simulink library "FSCtrl_cl"  (R2020a)
settings: Solver=VariableStepAuto  StartTime=0.0  StopTime=10.0  RelTol=1e-3
undefined symbols (not defined in the file or in its folder): a, env, FLIGHTCONTROLLER, fltCtrl, initializeBussesFromBlock, pthCtrl1, pthCtrl2, slfCtrl, thr, vhcl, wnch
libraries: simulink x22, angleBtw2Vecs_ul x6, filteredPIDController_ul x5, velocityAngle_ul x4, ctrlAllocMatrix_cl x3, filteredPIDControllerAWGS_ul x3, eulAng2RotMat_ul x3, vrlib x3, alphaBeta_ul x3, gnd2TanRotation_ul x3, pathGeometry_ul x3, filteredPIDControllerAW_ul x2
(part 2 of 3)

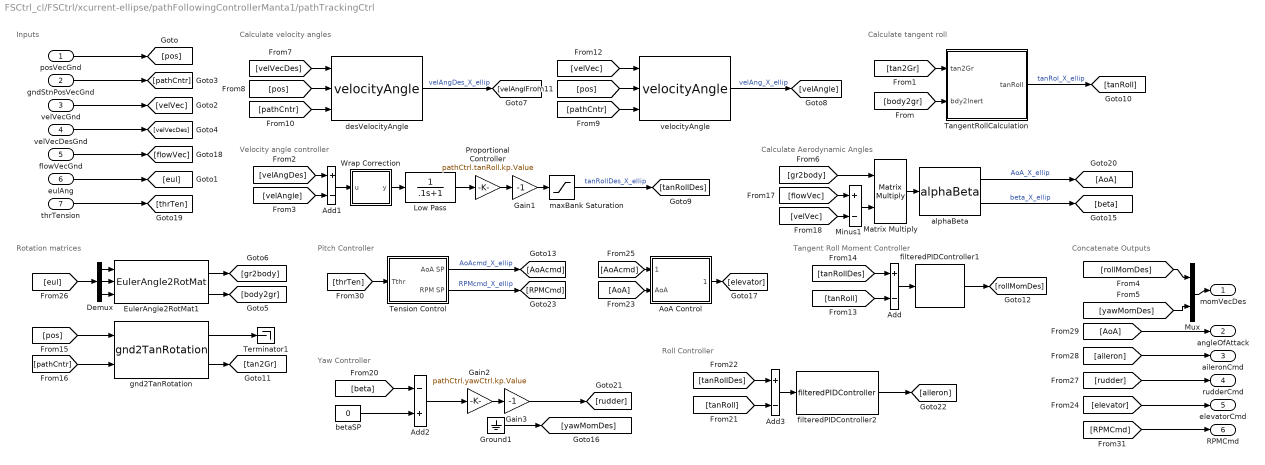
== system FSCtrl_cl/FSCtrl/xcurrent-ellipse/pathFollowingControllerManta1/pathTrackingCtrl ==
  note: Pitch Controller
  note: Calculate Aerodynamic Angles
  note: Yaw Controller
  note: Concatenate Outputs
  note: Tangent Roll Moment Controller
  note: Calculate tangent roll
  note: Calculate velocity angles
  note: Rotation matrices
  note: Inputs
  note: Velocity angle controller
  note: Roll Controller
  posVecGnd : Inport
  gndStnPosVecGnd : Inport  Port=2
  velVecGnd : Inport  Port=3
  velVecDesGnd : Inport  Port=4
  flowVecGnd : Inport  Port=5
  eulAng : Inport  Port=6
  thrTension : Inport  Port=7
  Add : Sum  Inputs=+-
  Add1 : Sum  Inputs=+-
  Add2 : Sum  Inputs=-+
  Add3 : Sum  Inputs=+-
  AoA Control : Subsystem
  Demux : Demux  Outputs=3
  EulerAngle2RotMat1 : eulAng2RotMat_ul/EulerAngle2RotMat  SystemSampleTime=-1  Latency=0  AutoFrameSizeCalculation=off
  Gain1 : Gain  Gain=-1
  Gain2 : Gain  Gain=pathCtrl.yawCtrl.kp.Value
  Gain3 : Gain  Gain=-1
  Ground1 : Ground
  Low Pass : TransferFcn  Denominator=[.1 1]
  Matrix Multiply : Product  Multiplication=Matrix(*)
  Minus1 : Sum  Inputs=+-
  Mux : Mux  Inputs=2
  Proportional Controller : Gain  Gain=pathCtrl.tanRoll.kp.Value
  TangentRollCalculation : Subsystem
  Tension Control : Subsystem
  Terminator1 : Terminator
  Wrap Correction : Subsystem
  alphaBeta : alphaBeta_ul/alphaBeta  SystemSampleTime=-1  Latency=0  AutoFrameSizeCalculation=off
  betaSP : Constant  Value=0
  desVelocityAngle : velocityAngle_ul/velocityAngle  SystemSampleTime=-1  Latency=0  AutoFrameSizeCalculation=off
  filteredPIDController1 : filteredPIDController_ul/filteredPIDController  kp=pathCtrl.rollMoment.kp.Value  ki=0  kd=pathCtrl.rollMoment.kd.Value  Value=pathCtrl.rollMoment.tau.Value  externalReset=none
  filteredPIDController2 : filteredPIDController_ul/filteredPIDController  kp=pathCtrl.rollCtrl.kp.Value  ki=pathCtrl.rollCtrl.ki.Value  kd=pathCtrl.rollCtrl.kd.Value  Value=pathCtrl.rollCtrl.tau.Value  externalReset=none
  gnd2TanRotation : gnd2TanRotation_ul/gnd2TanRotation  SystemSampleTime=-1  Latency=0  AutoFrameSizeCalculation=off
  maxBank Saturation : Saturate  UpperLimit=pathCtrl.maxBank.upperLimit.Value  LowerLimit=pathCtrl.maxBank.lowerLimit.Value
  velocityAngle : velocityAngle_ul/velocityAngle  SystemSampleTime=-1  Latency=0  AutoFrameSizeCalculation=off
  momVecDes : Outport  VectorParamsAs1DForOutWhenUnconnected=off
  angleOfAttack : Outport  Port=2  VectorParamsAs1DForOutWhenUnconnected=off
  aileronCmd : Outport  Port=3  VectorParamsAs1DForOutWhenUnconnected=off
  rudderCmd : Outport  Port=4  VectorParamsAs1DForOutWhenUnconnected=off
  elevatorCmd : Outport  Port=5  VectorParamsAs1DForOutWhenUnconnected=off
  RPMCmd : Outport  Port=6  VectorParamsAs1DForOutWhenUnconnected=off
  wires:
  Ground1/1 -> [yawMomDes]
  Low Pass/1 -> Proportional Controller/1
  Wrap Correction/1(y) -> Low Pass/1
  posVecGnd/1 -> [pos]
  velVecGnd/1 -> [velVec]
  Add/1 -> filteredPIDController1/1
  Proportional Controller/1 -> Gain1/1
  Gain1/1 -> maxBank Saturation/1
  maxBank Saturation/1 -> [tanRollDes]  "tanRollDes_X_ellip"
  Add1/1 -> Wrap Correction/1(u)
  flowVecGnd/1 -> [flowVec]
  [tan2Gr] -> TangentRollCalculation/1(tan2Gr)
  TangentRollCalculation/1(tanRoll) -> [tanRoll]  "tanRol_X_ellip"
  filteredPIDController1/1 -> [rollMomDes]
  Gain2/1 -> Gain3/1
  Minus1/1 -> Matrix Multiply/2
  [velVec] -> Minus1/2
  [flowVec] -> Minus1/1
  Demux/3 -> EulerAngle2RotMat1/3
  Demux/1 -> EulerAngle2RotMat1/1
  Demux/2 -> EulerAngle2RotMat1/2
  EulerAngle2RotMat1/2 -> [body2gr]
  EulerAngle2RotMat1/1 -> [gr2body]
  [body2gr] -> TangentRollCalculation/2(bdy2Inert)
  [gr2body] -> Matrix Multiply/1
  Matrix Multiply/1 -> alphaBeta/1
  alphaBeta/2 -> [beta]  "beta_X_ellip"
  Add2/1 -> Gain2/1
  Mux/1 -> momVecDes/1
  [yawMomDes] -> Mux/2
  gndStnPosVecGnd/1 -> [pathCntr]
  velVecDesGnd/1 -> [velVecDes]
  desVelocityAngle/1 -> [velAngDes]  "velAngDes_X_ellip"
  velocityAngle/1 -> [velAngle]  "velAng_X_ellip"
  [velAngDes] -> Add1/1
  [velAngle] -> Add1/2
  [velVecDes] -> desVelocityAngle/1
  [pos] -> desVelocityAngle/2
  [pathCntr] -> desVelocityAngle/3
  [velVec] -> velocityAngle/1
  [tanRoll] -> Add/2
  [tanRollDes] -> Add/1
  [pos] -> gnd2TanRotation/1
  [pathCntr] -> gnd2TanRotation/2
  gnd2TanRotation/2 -> [tan2Gr]
  gnd2TanRotation/1 -> Terminator1/1
  [rollMomDes] -> Mux/1
  Tension Control/2(RPM SP) -> [RPMCmd]  "RPMcmd_X_ellip"
  AoA Control/1(elvCmd) -> [elevator]
  Tension Control/1(AoA SP) -> [AoAcmd]  "AoAcmd_X_ellip"
  [AoAcmd] -> AoA Control/1(AoA SP)
  [AoA] -> AoA Control/2(AoA)
  eulAng/1 -> [eul]
  thrTension/1 -> [thrTen]
  [eul] -> Demux/1
  [thrTen] -> Tension Control/1(Tthr)
  [pos] -> velocityAngle/2
  [pathCntr] -> velocityAngle/3
  alphaBeta/1 -> [AoA]  "AoA_X_ellip"
  Gain3/1 -> [rudder]
  [beta] -> Add2/1
  betaSP/1 -> Add2/2
  filteredPIDController2/1 -> [aileron]
  [AoA] -> angleOfAttack/1
  [aileron] -> aileronCmd/1
  [rudder] -> rudderCmd/1
  [elevator] -> elevatorCmd/1
  [tanRollDes] -> Add3/1
  [tanRoll] -> Add3/2
  Add3/1 -> filteredPIDController2/1
  [RPMCmd] -> RPMCmd/1

== system FSCtrl_cl/FSCtrl/xcurrent-lemOfBooth/pathFollowingControllerManta/Concatenation ==
  In1 : Inport
  Demux1 : Demux
  Gain : Gain  Gain=pathCtrl.rudderGain.Value
  Mux : Mux
  Out1 : Outport
  wires:
  In1/1 -> Demux1/1
  Mux/1 -> Out1/1
  Demux1/4 -> Gain/1
  Gain/1 -> Mux/4  "rudderCmd"
  Demux1/2 -> Mux/2  "starBrdCmd"
  Demux1/1 -> Mux/1  "portCmd"
  Demux1/3 -> Mux/3  "elevCmd"

== system FSCtrl_cl/FSCtrl/xcurrent-lemOfBooth/pathFollowingControllerManta/Lap Tracking ==
  pathParameter : Inport
  Add2 : Sum
  Compare To Constant1 : simulink/Logic and Bit Operations/Compare To Constant  relop=>=  const=10  OutDataTypeStr=boolean
  Compare To Constant3 : simulink/Logic and Bit Operations/Compare To Constant  relop=<=  const=0.1  OutDataTypeStr=boolean
  Compare To Constant4 : simulink/Logic and Bit Operations/Compare To Constant  relop=>=  const=0.9  OutDataTypeStr=boolean
  Data Type Conversion2 : DataTypeConversion  OutDataTypeStr=double
  Logical Operator1 : Logic  Inputs=4  AllPortsSameDT=off  OutDataTypeStr=boolean
  Memory : Memory  InitialCondition=false
  Memory3 : Memory
  Memory4 : Memory
  Subsystem : Subsystem
  stopwatch : stopwatch_ul/stopwatch  SystemSampleTime=-1  Latency=0  AutoFrameSizeCalculation=off
  lapNum : Outport  VectorParamsAs1DForOutWhenUnconnected=off
  rst : Outport  Port=2  VectorParamsAs1DForOutWhenUnconnected=off
  wires:
  Subsystem/1(realLap) -> Logical Operator1/3  "real"
  Compare To Constant1/1 -> Logical Operator1/4
  Memory/1 -> stopwatch/1, Subsystem/2(rst)
  stopwatch/1 -> Compare To Constant1/1
  pathParameter/1 -> Memory3/1, Compare To Constant3/1, Subsystem/1(S)
  Compare To Constant4/1 -> Logical Operator1/2
  Add2/1 -> Memory4/1, lapNum/1
  Memory4/1 -> Add2/2
  Logical Operator1/1 -> Memory/1, Data Type Conversion2/1, rst/1
  Data Type Conversion2/1 -> Add2/1
  Memory3/1 -> Compare To Constant4/1
  Compare To Constant3/1 -> Logical Operator1/1

== system FSCtrl_cl/FSCtrl/xcurrent-lemOfBooth/pathFollowingControllerManta/Subsystem ==
  posVecGnd : Inport
  Atan1 : Trigonometry  Operator=atan2
  Atan2 : Trigonometry  Operator=atan2
  Gain : Gain  Gain=180/pi
  Gain1 : Gain  Gain=180/pi
  Selector1 : Selector  InputPortWidth=3  IndexOptions=Index vector (dialog)  Indices=1  OutputSizes=1
  Selector2 : Selector  InputPortWidth=3  IndexOptions=Index vector (dialog)  Indices=[1 2]  OutputSizes=1
  Selector3 : Selector  InputPortWidth=3  IndexOptions=Index vector (dialog)  Indices=3  OutputSizes=1
  Selector4 : Selector  InputPortWidth=3  IndexOptions=Index vector (dialog)  Indices=2  OutputSizes=1
  Sqrt1 : Sqrt  SaturateOnIntegerOverflow=on
  Sqrt2 : Sqrt  SaturateOnIntegerOverflow=on
  Square1 : Math  Operator=square  SignedPower=on  SaturateOnIntegerOverflow=on
  Square2 : Math  Operator=square  SignedPower=on  SaturateOnIntegerOverflow=on
  Sum of Elements : Sum  Inputs=+
  Sum of Elements1 : Sum  Inputs=+
  elevationAngle : Outport
  azimuth Angle : Outport  Port=2
  wires:
  Gain1/1 -> azimuth Angle/1
  Selector4/1 -> Atan2/1
  Sqrt2/1 -> Atan2/2
  posVecGnd/1 -> Selector3/1, Selector2/1, Selector4/1, Selector1/1
  Selector1/1 -> Square2/1
  Sum of Elements1/1 -> Sqrt2/1
  Square2/1 -> Sum of Elements1/1
  Atan2/1 -> Gain1/1
  Gain/1 -> elevationAngle/1
  Selector2/1 -> Square1/1
  Atan1/1 -> Gain/1
  Sum of Elements/1 -> Sqrt1/1
  Selector3/1 -> Atan1/1
  Square1/1 -> Sum of Elements/1
  Sqrt1/1 -> Atan1/2

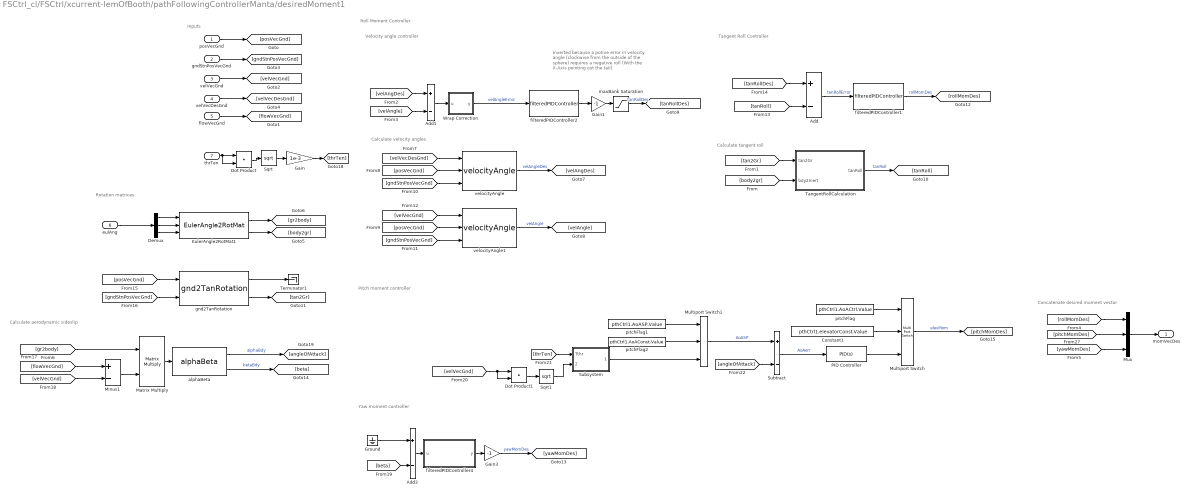
== system FSCtrl_cl/FSCtrl/xcurrent-lemOfBooth/pathFollowingControllerManta/desiredMoment1 ==
  note: Roll Moment Controller
  note: Calculate aerodynamic sideslip
  note: Concatenate desired moment vector
  note: Tangent Roll Controller
  note: Calculate tangent roll
  note: Calculate velocity angles
  note: Rotation matrices
  note: Inputs
  note: Velocity angle controller
  note: Inverted because a potive error
      | in velocity angle (clockwise from the
      | outside of the sphere) requires a negative
      | roll (With the X-Axis pointing out the tail)
  note: Pitch moment controller
  note: Yaw moment controller
  posVecGnd : Inport
  gndStnPosVecGnd : Inport  Port=2
  velVecGnd : Inport  Port=3
  velVecDesGnd : Inport  Port=4
  flowVecGnd : Inport  Port=5
  eulAng : Inport  Port=6
  thrTen : Inport  Port=7
  Add : Sum  Inputs=+-
  Add1 : Sum  Inputs=+-
  Add3 : Sum  Inputs=+-
  Constant1 : Constant  Value=pthCtrl1.elevatorConst.Value
  Demux : Demux  Outputs=3
  Dot Product : DotProduct  InputSameDT=on  OutDataTypeStr=Inherit: Inherit via internal rule
  Dot Product1 : DotProduct  InputSameDT=on  OutDataTypeStr=Inherit: Inherit via internal rule
  EulerAngle2RotMat1 : eulAng2RotMat_ul/EulerAngle2RotMat  SystemSampleTime=-1  Latency=0  AutoFrameSizeCalculation=off
  Gain : Gain  Gain=1e-3
  Gain1 : Gain  Gain=-1
  Gain3 : Gain  Gain=-1
  Ground : Ground
  Matrix Multiply : Product  Multiplication=Matrix(*)
  Minus1 : Sum  Inputs=+-
  Multiport Switch : MultiPortSwitch  DataPortOrder=Specify indices  Inputs=2  DataPortIndices={0,1}
  Multiport Switch1 : MultiPortSwitch  DataPortOrder=Specify indices  Inputs=2  DataPortIndices={0,1}
  Mux : Mux  Inputs=3
  PID Controller : simulink/Continuous/PID Controller  Controller=PID  Form=Parallel  TimeDomain=Continuous-time  UseExternalTs=off  SampleTime=-1  IntegratorMethod=Forward Euler  FilterMethod=Forward Euler  ControllerParametersSource=internal  P=pthCtrl1.pitchMoment.kp.Value  I=pthCtrl1.pitchMoment.ki.Value  D=pthCtrl1.pitchMoment.kd.Value  UseFilter=on  N=pthCtrl1.pitchMoment.tau.Value  TunerSelectOption=Transfer Function Based (PID Tuner App)  InitialConditionSource=internal  InitialConditionForIntegrator=0  InitialConditionForFilter=0  DifferentiatorICPrevScaledInput=0  ExternalReset=none  TrackingMode=off  Kt=1  LimitOutput=off  UpperSaturationLimit=inf  LowerSaturationLimit=-100  LinearizeAsGain=on  AntiWindupMode=clamping  Kb=1  POutMin=[]  POutMax=[]  IOutMin=[]  IOutMax=[]  DOutMin=[]  DOutMax=[]  NOutMin=[]  NOutMax=[]  SumOutMin=[]  SumOutMax=[]  SaturationOutMin=[]  SaturationOutMax=[]  PParamMin=[]  PParamMax=[]  IParamMin=[]  IParamMax=[]  DParamMin=[]  DParamMax=[]  NParamMin=[]  NParamMax=[]  KbParamMin=[]  KbParamMax=[]  KtParamMin=[]  KtParamMax=[]  KbOutMin=[]  KbOutMax=[]  KtOutMin=[]  KtOutMax=[]  IntegratorOutMin=[]  IntegratorOutMax=[]  FilterOutMin=[]  FilterOutMax=[]  SumI1OutMin=[]  SumI1OutMax=[]  SumI2OutMin=[]  SumI2OutMax=[]  SumI3OutMin=[]  SumI3OutMax=[]  SumI4OutMin=[]  SumI4OutMax=[]  SumDOutMin=[]  SumDOutMax=[]  DifferentiatorOutMin=[]  DifferentiatorOutMax=[]  FilterDiffOutCoefMin=[]  FilterDiffOutCoefMax=[]  ReciprocalOutMin=[]  ReciprocalOutMax=[]  SumDenOutMin=[]  SumDenOutMax=[]  SumNumOutMin=[]  SumNumOutMax=[]  DivideOutMin=[]  DivideOutMax=[]  UdiffTsProdOutMin=[]  UdiffTsProdOutMax=[]  NTsProdOutMin=[]  NTsProdOutMax=[]  UintegralTsProdOutMin=[]  UintegralTsProdOutMax=[]  UngainTsProdOutMin=[]  UngainTsProdOutMax=[]  IntegratorContinuousStateAttributes=''  IntegratorStateMustResolveToSignalObject=off  IntegratorRTWStateStorageClass=Auto  FilterContinuousStateAttributes=''  FilterStateMustResolveToSignalObject=off  FilterRTWStateStorageClass=Auto  ParallelPVariant=InternalParameters  IdealPVariant=Disabled  IVariant=InternalParameters  DVariant=InternalParameters  IntegratorVariant=Continuous  SatVariant=Disabled  AWVariant=Passthrough  PCopyVariant=Disabled  TRVariant=Disabled  FdbkBlocksVariant=Forward  IdealPFdbkVariant=Disabled  SatFdbkVariant=Disabled  DerivativeFilterVariant=ContFilter  NVariant=InternalParameters  NCopyVariant=Disabled  FilterICVariant=InternalICsFilter  IntegratorICVariant=InternalICs  ExternalResetVariant=Disabled  TRSumVariant=Passthrough  SumFdbkVariant=Disabled  SumVariant=Sum_PID  TsampFilterVariant=InternalTs  TsampNgainVariant=Passthrough  TsampIntegralVariant=Passthrough
  Sqrt : Sqrt  SaturateOnIntegerOverflow=on
  Sqrt1 : Sqrt  SaturateOnIntegerOverflow=on
  Subsystem : Subsystem
  Subtract : Sum  Inputs=+-
  TangentRollCalculation : Subsystem
  Terminator1 : Terminator
  Wrap Correction : Subsystem
  alphaBeta : alphaBeta_ul/alphaBeta  SystemSampleTime=-1  Latency=0  AutoFrameSizeCalculation=off
  filteredPIDController1 : filteredPIDController_ul/filteredPIDController  kp=pathCtrl.rollMoment.kp.Value  ki=0  kd=pathCtrl.rollMoment.kd.Value  Value=pathCtrl.rollMoment.tau.Value  externalReset=none
  filteredPIDController2 : filteredPIDController_ul/filteredPIDController  kp=pathCtrl.tanRoll.kp.Value  ki=pathCtrl.tanRoll.ki.Value  kd=pathCtrl.tanRoll.kd.Value  Value=pathCtrl.tanRoll.tau.Value  externalReset=none
  filteredPIDController4 : Subsystem  mask{kp=pthCtrl1.yawMoment.kp.Value, ki=0, kd=pathCtrl.yawMoment.kd.Value, Value=pathCtrl.yawMoment.tau.Value, externalReset=none}
      mask prompts: kp "Proportional Gain, kp"; ki "Integral Gain, ki"; kd "Derivative Gain, kd"; Value "Time Constant, s"; externalReset "External reset:"
      mask init:
      | initfcn
      mask TypeOptions kp: kp/Gain
      mask TypeOptions ki: ki/Gain
      mask TypeOptions kd: kd/Gain
      mask TypeOptions Value: tau/Value
      mask TypeOptions externalReset: none | rising | falling | either | level | level hold
  gnd2TanRotation : gnd2TanRotation_ul/gnd2TanRotation  SystemSampleTime=-1  Latency=0  AutoFrameSizeCalculation=off
  maxBank Saturation : Saturate  UpperLimit=pathCtrl.maxBank.upperLimit.Value  LowerLimit=pathCtrl.maxBank.lowerLimit.Value
  pitchFlag : Constant  Value=pthCtrl1.AoACtrl.Value
  pitchFlag1 : Constant  Value=pthCtrl1.AoASP.Value
  pitchFlag2 : Constant  Value=pthCtrl1.AoAConst.Value
  velocityAngle : velocityAngle_ul/velocityAngle  SystemSampleTime=-1  Latency=0  AutoFrameSizeCalculation=off
  velocityAngle1 : velocityAngle_ul/velocityAngle  SystemSampleTime=-1  Latency=0  AutoFrameSizeCalculation=off
  momVecDes : Outport  VectorParamsAs1DForOutWhenUnconnected=off
  wires:
  filteredPIDController1/1 -> [rollMomDes]  "rollMomDes"
  [rollMomDes] -> Mux/1
  Wrap Correction/1(y) -> filteredPIDController2/1  "velAngleError"
  posVecGnd/1 -> [posVecGnd]
  velVecGnd/1 -> [velVecGnd]
  Add/1 -> filteredPIDController1/1  "tanRollError"
  Gain1/1 -> maxBank Saturation/1
  maxBank Saturation/1 -> [tanRollDes]  "tanRollDes"
  Add1/1 -> Wrap Correction/1(u)
  flowVecGnd/1 -> [flowVecGnd]
  [tan2Gr] -> TangentRollCalculation/1(tan2Gr)
  TangentRollCalculation/1(tanRoll) -> [tanRoll]  "tanRoll"
  Minus1/1 -> Matrix Multiply/2
  [velVecGnd] -> Minus1/2
  [flowVecGnd] -> Minus1/1
  eulAng/1 -> Demux/1
  Demux/2 -> EulerAngle2RotMat1/2
  EulerAngle2RotMat1/2 -> [body2gr]
  EulerAngle2RotMat1/1 -> [gr2body]
  [body2gr] -> TangentRollCalculation/2(bdy2Inert)
  [gr2body] -> Matrix Multiply/1
  Matrix Multiply/1 -> alphaBeta/1
  alphaBeta/2 -> [beta]  "betaBdy"
  alphaBeta/1 -> [angleOfAttack]  "alphaBdy"
  gndStnPosVecGnd/1 -> [gndStnPosVecGnd]
  velVecDesGnd/1 -> [velVecDesGnd]
  velocityAngle/1 -> [velAngDes]  "velAngleDes"
  velocityAngle1/1 -> [velAngle]  "velAngle"
  [velAngDes] -> Add1/1
  [velAngle] -> Add1/2
  [velVecDesGnd] -> velocityAngle/1
  [posVecGnd] -> velocityAngle/2
  [posVecGnd] -> velocityAngle1/2
  [gndStnPosVecGnd] -> velocityAngle/3
  [gndStnPosVecGnd] -> velocityAngle1/3
  [velVecGnd] -> velocityAngle1/1
  [tanRoll] -> Add/2
  [tanRollDes] -> Add/1
  [posVecGnd] -> gnd2TanRotation/1
  [gndStnPosVecGnd] -> gnd2TanRotation/2
  gnd2TanRotation/2 -> [tan2Gr]
  gnd2TanRotation/1 -> Terminator1/1
  [yawMomDes] -> Mux/3
  filteredPIDController2/1 -> Gain1/1
  [beta] -> Add3/2
  Ground/1 -> Add3/1
  Add3/1 -> filteredPIDController4/1(u)
  filteredPIDController4/1(y) -> Gain3/1
  Subsystem/1(AoA SP) -> Multiport Switch1/3
  [thrTen] -> Subsystem/1(Tthr)
  pitchFlag1/1 -> Multiport Switch1/1
  pitchFlag2/1 -> Multiport Switch1/2
  [pitchMomDes] -> Mux/2
  Gain3/1 -> [yawMomDes]  "yawMomDes"
  Multiport Switch/1 -> [pitchMomDes]  "elevMom"
  pitchFlag/1 -> Multiport Switch/1
  [angleOfAttack] -> Subtract/2
  Constant1/1 -> Multiport Switch/2
  PID Controller/1 -> Multiport Switch/3
  Subtract/1 -> PID Controller/1  "AoAerr"
  thrTen/1 -> Dot Product/2, Dot Product/1
  Sqrt/1 -> Gain/1
  Dot Product/1 -> Sqrt/1
  Gain/1 -> [thrTen]
  [velVecGnd] -> Dot Product1/2, Dot Product1/1
  Sqrt1/1 -> Subsystem/2(vAppSqr)
  Dot Product1/1 -> Sqrt1/1
  Demux/1 -> EulerAngle2RotMat1/1
  Demux/3 -> EulerAngle2RotMat1/3
  Mux/1 -> momVecDes/1
  Multiport Switch1/1 -> Subtract/1  "AoASP"

== system FSCtrl_cl/FSCtrl/non-xcurrent/LaRController/desiredMoment/TangentRollCalculation ==
  note: Angle between body X and tangent Z
  note: Inverted because the right wing
      | being <90deg from Local down
      | is a negative roll about the +X axis
  note: Angle between body Y and tangent Z
  note: Measuring tangent roll as the opposite
      | of the angle between the Body Y axis
      | and the tangent plane
  tan2Gr : Inport
  bdy2Inert : Inport  Port=2
  Constant1 : Constant  Value=pi/2
  Constant2 : Constant  Value=pi/2
  Constant3 : Constant  Value=[0 1 0]'
  Constant4 : Constant  Value=[0 0 1]'
  Constant5 : Constant  Value=[1 0 0]'
  Constant6 : Constant  Value=[0 0 1]'
  Gain : Gain  Gain=-1
  Matrix Multiply{,1..3} (4 alike) : Product  Multiplication=Matrix(*)
  Subtract : Sum  Inputs=+-
  Subtract1 : Sum  Inputs=+-
  Terminator : Terminator
  angleBtw2DVecs : angleBtw2Vecs_ul/angleBtw2DVecs  SystemSampleTime=-1  Latency=0  AutoFrameSizeCalculation=off
  angleBtw2DVecs1 : Subsystem
  tanRoll : Outport  VectorParamsAs1DForOutWhenUnconnected=off
  wires:
  Constant5/1 -> Matrix Multiply2/2
  angleBtw2DVecs1/1(angle) -> Subtract1/2
  Constant1/1 -> Subtract1/1
  Matrix Multiply3/1 -> angleBtw2DVecs1/1(vec1)
  Constant6/1 -> Matrix Multiply3/2
  Matrix Multiply2/1 -> angleBtw2DVecs1/2(vec2)
  tan2Gr/1 -> Matrix Multiply1/1, Matrix Multiply3/1
  Subtract1/1 -> Terminator/1  "tanPitch"
  bdy2Inert/1 -> Matrix Multiply/1, Matrix Multiply2/1
  Gain/1 -> tanRoll/1  "tanRoll"
  Subtract/1 -> Gain/1
  Matrix Multiply/1 -> angleBtw2DVecs/2
  Constant4/1 -> Matrix Multiply1/2
  Matrix Multiply1/1 -> angleBtw2DVecs/1
  Constant2/1 -> Subtract/1
  angleBtw2DVecs/1 -> Subtract/2
  Constant3/1 -> Matrix Multiply/2

== system FSCtrl_cl/FSCtrl/non-xcurrent/LaRController/winchController/vectorMagnitude ==
  Vec : Inport
  Reshape4 : Reshape
  Sqrt : Sqrt  SaturateOnIntegerOverflow=on
  Square : Math  Operator=square  SaturateOnIntegerOverflow=on
  Sum of Elements : Sum  Inputs=+
  Mag : Outport
  wires:
  Reshape4/1 -> Mag/1
  Vec/1 -> Square/1
  Sum of Elements/1 -> Sqrt/1
  Square/1 -> Sum of Elements/1
  Sqrt/1 -> Reshape4/1

== system FSCtrl_cl/FSCtrl/xcurrent-ellipse/pathFollowingControllerManta1/Lap Tracking/Subsystem ==
  note: this may have issues when it starts up after a hiatus for a multicycle spool in
      | Hopefully, it will work because the reasonable spooling ranges are already set
  S : Inport
  rst : Inport  Port=2
  AND : Logic  AllPortsSameDT=off  OutDataTypeStr=boolean
  Add : Sum
  Cast To Double : DataTypeConversion  OutDataTypeStr=double
  Compare To Constant : simulink/Logic and Bit Operations/Compare To Constant  relop=>=  const=.99  OutDataTypeStr=boolean
  Compare To Constant1 : simulink/Logic and Bit Operations/Compare To Constant  relop=<=  const=.01  OutDataTypeStr=boolean
  Divide : Product  Inputs=**
  Divide1 : Product  Inputs=**
  Gain : Gain  Gain=-1
  Max : MinMax  Function=max  Inputs=2
  Max1 : MinMax  Inputs=2
  One : Constant  OutDataTypeStr=Inherit: Inherit via back propagation
  Power : Math  Operator=pow  SaturateOnIntegerOverflow=on
  Power1 : Math  Operator=pow  SaturateOnIntegerOverflow=on
  memoryIC1 : Memory  InitialCondition=1
  memoryIC=0 : Memory
  memoryIC=1 : Memory  InitialCondition=1
  realLap : Outport
  wires:
  memoryIC1/1 -> Power/1
  memoryIC=1/1 -> Power1/1
  [zeroIfReset] -> Power1/2
  memoryIC=0/1 -> Divide1/1
  Divide1/1 -> Max/2
  [zeroIfReset] -> Divide1/2
  [zeroIfReset] -> Power/2
  [zeroIfReset] -> Divide/2
  AND/1 -> realLap/1
  Compare To Constant1/1 -> AND/2
  Compare To Constant/1 -> AND/1
  Cast To Double/1 -> Gain/1
  Power1/1 -> Max1/2
  Power/1 -> Max1/1
  Max/1 -> Compare To Constant/1, memoryIC=0/1
  Divide/1 -> Max/1
  One/1 -> Add/2
  Add/1 -> [zeroIfReset]
  Gain/1 -> Add/1
  S/1 -> memoryIC1/1, Divide/1
  rst/1 -> Cast To Double/1
  Max1/1 -> memoryIC=1/1, Compare To Constant1/1

== system FSCtrl_cl/FSCtrl/xcurrent-ellipse/pathFollowingControllerManta1/courseFollowManta/GoldenSectionPathSearch ==
  lastKnownS : Inport
  pathParams : Inport  Port=2
  currentPos : Inport  Port=3
  pathCntr : Inport  Port=4
  From11 : From  Commented=on  GotoTag=geomParams
  From27 : From  Commented=on  GotoTag=pathCntr
  From28 : From  Commented=on  GotoTag=pos
  From30 : From  Commented=on  GotoTag=sPrev
  GoldenSectionMATLAB : MATLAB Function  Commented=on  TreatAsAtomicUnit=on  mask{geomFunc=pathCtrl, searchWidth=0.1, pathVarTol=1e-5}
  GoldenSectionSimulink : Subsystem
  Goto1 : Goto  Commented=on  GotoTag=sStar
  sStar : Outport  InitialOutput=pathCtrl.initPathVar.Value  VectorParamsAs1DForOutWhenUnconnected=off
  wires:
  GoldenSectionSimulink/1(Out1) -> [sStar]
  [sPrev] -> GoldenSectionSimulink/4(sPrev)
  [pathCntr] -> GoldenSectionSimulink/3(cntrPtPosVec)
  [geomParams] -> GoldenSectionSimulink/2(geomParams)
  [pos] -> GoldenSectionSimulink/1(posVecGnd)
  [sStar] -> sStar/1
  lastKnownS/1 -> [sPrev]
  From27/1 -> GoldenSectionMATLAB/3(pathCntrPosVecGnd)
  From30/1 -> GoldenSectionMATLAB/2(sPrev)
  From28/1 -> GoldenSectionMATLAB/1(posVec)
  From11/1 -> GoldenSectionMATLAB/4(geomParams)
  GoldenSectionMATLAB/1(sNext) -> Goto1/1
  pathCntr/1 -> [pathCntr]
  pathParams/1 -> [geomParams]
  currentPos/1 -> [pos]

== system FSCtrl_cl/FSCtrl/xcurrent-ellipse/pathFollowingControllerManta1/courseFollowManta/Overwrite Radius ==
  note: subsystem overwrites the 5th basis parameter with the current radius
      | so that the downstream blocks calculate the path geomatry at the current radius.
  pathParamsIn : Inport
  positionVec : Inport  Port=2
  gndStnPos : Inport  Port=3
  Add : Sum  Inputs=+-
  Assignment : Assignment  NumberOfDimensions=2  DiagnosticForDimensions=Warning  IndexOptions=Index vector (dialog),Assign all  Indices=5,5  OutputSizes=1,1
  Dot Product : DotProduct  InputSameDT=on  OutDataTypeStr=Inherit: Inherit via internal rule
  Sqrt : Sqrt  SaturateOnIntegerOverflow=on
  pathParamsOut : Outport  VectorParamsAs1DForOutWhenUnconnected=off
  wires:
  gndStnPos/1 -> Add/2
  positionVec/1 -> Add/1
  pathParamsIn/1 -> Assignment/1
  Sqrt/1 -> Assignment/2
  Assignment/1 -> pathParamsOut/1
  Dot Product/1 -> Sqrt/1
  Add/1 -> Dot Product/1, Dot Product/2

== system FSCtrl_cl/FSCtrl/xcurrent-ellipse/pathFollowingControllerManta1/courseFollowManta/saturatedWeightedAverage ==
  note: 0 if error=0
      | 1 if error>=upper_lim
  note: from mask
  note: errorVar must be positive
  "errorVar " : Inport
  tangVector : Inport  Port=2
  "perpVector " : Inport  Port=3
  Add : Sum  Commented=on  Inputs=+-
  Add1 : Sum  Commented=on
  Add2 : Sum  Inputs=+-
  Add3 : Sum
  Constant : Constant  Value=error_upper_lim
  Constant1 : Constant  Commented=on  Value=a
  Constant2 : Constant  Commented=on
  Constant4 : Constant
  Divide : Product  Inputs=*/
  Exp : Math  Commented=on  SignedPower=on  SaturateOnIntegerOverflow=on
  From : From  Commented=on  GotoTag=errorVar
  From1 : From  Commented=on  GotoTag=perpVec
  From2 : From  Commented=on  GotoTag=tangVec
  Gain : Gain  Commented=on  Gain=-1
  Multiply : Product  Commented=on
  Multiply1 : Product  Commented=on
  Multiply2 : Product  Commented=on
  Multiply3 : Product
  Multiply5 : Product
  Saturation : Saturate  UpperLimit=1  LowerLimit=0
  "velVectorDes " : Outport  VectorParamsAs1DForOutWhenUnconnected=off
  wires:
  tangVector/1 -> [tangVector]
  Constant1/1 -> Gain/1
  Gain/1 -> Multiply1/1
  Multiply1/1 -> Exp/1
  Exp/1 -> Multiply/1, Add/2  "e^(-a*errorVar) 0 if error=inf 1 if error=0"
  Constant2/1 -> Add/1
  Add/1 -> Multiply2/1  "1-e^(-a*errorVar) 0 if error=0 1 if error=inf"
  "errorVar "/1 -> [errorVar]
  "perpVector "/1 -> [perpVector]
  From/1 -> Multiply1/2
  Multiply2/1 -> Add1/1
  Multiply/1 -> Add1/2
  From1/1 -> Multiply2/2
  From2/1 -> Multiply/2
  Constant4/1 -> Add2/1
  Saturation/1 -> Multiply3/1, Add2/2
  Add3/1 -> "velVectorDes "/1
  Multiply3/1 -> Add3/2
  Multiply5/1 -> Add3/1
  Add2/1 -> Multiply5/1  "0 if error>=upper_lim 1 if error=inf"
  [errorVar] -> Divide/1
  Constant/1 -> Divide/2
  Divide/1 -> Saturation/1
  [tangVector] -> Multiply5/2
  [perpVector] -> Multiply3/2

== system FSCtrl_cl/FSCtrl/xcurrent-ellipse/pathFollowingControllerManta1/pathTrackingCtrl/AoA Control ==
  AoA SP : Inport
  AoA : Inport  Port=2
  Constant1 : Constant  Value=pathCtrl.elevatorConst.Value
  Constant3 : Constant  Value=pathCtrl.elevCtrl.kp.Value
  Constant4 : Constant  Value=pathCtrl.elevCtrl.ki.Value
  Constant5 : Constant  Value=pathCtrl.elevCtrl.kd.Value
  Constant6 : Constant  Value=pathCtrl.elevCtrl.tau.Value
  Multiport Switch : MultiPortSwitch  DataPortOrder=Specify indices  Inputs=2  DataPortIndices={0,1}
  Mux : Mux
  Saturation : Saturate  UpperLimit=pathCtrl.elevCtrlMax.upperLimit.Value  LowerLimit=pathCtrl.elevCtrlMax.lowerLimit.Value
  Subtract : Sum  Inputs=-+
  filteredPIDControllerAWGS : filteredPIDControllerAWGS_ul/filteredPIDControllerAWGS  cmax=pathCtrl.elevCtrlMax.upperLimit.Value  cmin=pathCtrl.elevCtrlMax.lowerLimit.Value
  pitchFlag : Constant  Value=pathCtrl.AoACtrl.Value
  elvCmd : Outport
  wires:
  Constant6/1 -> Mux/4
  Constant5/1 -> Mux/3
  Constant4/1 -> Mux/2
  Constant3/1 -> Mux/1
  Mux/1 -> [gains]
  [gains] -> filteredPIDControllerAWGS/2
  filteredPIDControllerAWGS/1 -> Multiport Switch/3
  Subtract/1 -> filteredPIDControllerAWGS/1
  Saturation/1 -> elvCmd/1
  Multiport Switch/1 -> Saturation/1
  AoA SP/1 -> Subtract/1
  pitchFlag/1 -> Multiport Switch/1
  Constant1/1 -> Multiport Switch/2
  AoA/1 -> Subtract/2

== system FSCtrl_cl/FSCtrl/xcurrent-ellipse/pathFollowingControllerManta1/pathTrackingCtrl/TangentRollCalculation ==
  note: Measuring tangent roll as the opposite
      | of the angle between the Body Y axis
      | and the tangent plane
  note: Angle between body Y and tangent Z
  note: Inverted because the right wing
      | being <90deg from Local down
      | is a negative roll about the +X axis
  note: Angle between body X and tangent Z
  tan2Gr : Inport
  bdy2Inert : Inport  Port=2
  Constant1 : Constant  Value=pi/2
  Constant2 : Constant  Value=pi/2
  Constant3 : Constant  Value=[0 1 0]'
  Constant4 : Constant  Value=[0 0 1]'
  Constant5 : Constant  Value=[1 0 0]'
  Constant6 : Constant  Value=[0 0 1]'
  Gain : Gain  Gain=-1
  Matrix Multiply{,1..3} (4 alike) : Product  Multiplication=Matrix(*)
  Subtract : Sum  Inputs=+-
  Subtract1 : Sum  Inputs=+-
  Terminator : Terminator
  angleBtw2DVecs : angleBtw2Vecs_ul/angleBtw2DVecs  SystemSampleTime=-1  Latency=0  AutoFrameSizeCalculation=off
  angleBtw2DVecs1 : Subsystem
  tanRoll : Outport  VectorParamsAs1DForOutWhenUnconnected=off
  wires:
  Subtract/1 -> Gain/1
  Constant3/1 -> Matrix Multiply/2
  angleBtw2DVecs/1 -> Subtract/2
  Constant2/1 -> Subtract/1
  Matrix Multiply1/1 -> angleBtw2DVecs/1
  Constant4/1 -> Matrix Multiply1/2
  Matrix Multiply/1 -> angleBtw2DVecs/2
  Gain/1 -> tanRoll/1  "tanRoll"
  bdy2Inert/1 -> Matrix Multiply2/1, Matrix Multiply/1
  Subtract1/1 -> Terminator/1  "tanPitch"
  tan2Gr/1 -> Matrix Multiply3/1, Matrix Multiply1/1
  Matrix Multiply2/1 -> angleBtw2DVecs1/2(vec2)
  Constant6/1 -> Matrix Multiply3/2
  Matrix Multiply3/1 -> angleBtw2DVecs1/1(vec1)
  Constant1/1 -> Subtract1/1
  angleBtw2DVecs1/1(angle) -> Subtract1/2
  Constant5/1 -> Matrix Multiply2/2

== system FSCtrl_cl/FSCtrl/xcurrent-ellipse/pathFollowingControllerManta1/pathTrackingCtrl/Tension Control ==
  Tthr : Inport
  Compare To Constant : simulink/Logic and Bit Operations/Compare To Constant  relop===  const=1  OutDataTypeStr=boolean
  Constant : Constant  Value=pathCtrl.TmaxCtrl.Value
  Multiport Switch2 : MultiPortSwitch  DataPortOrder=Specify indices  Inputs=2  DataPortIndices={0,1}
  pitchFlag1 : Constant  Value=pathCtrl.AoASP.Value
  pitchFlag2 : Constant  Value=pathCtrl.AoAConst.Value
  tensionLimitAoA : tensionLimitAoA_cl/tensionLimitAoA  SystemSampleTime=-1  VariantControl=pathCtrl.TmaxCtrl.Value == 1  Latency=0  AutoFrameSizeCalculation=off
  AoA SP : Outport
  RPM SP : Outport  Port=2
  wires:
  [RPM1] -> RPM SP/1
  Compare To Constant/1 -> tensionLimitAoA/Enable
  Constant/1 -> Compare To Constant/1
  Tthr/1 -> tensionLimitAoA/1
  tensionLimitAoA/1 -> [AoA1]
  tensionLimitAoA/2 -> [RPM1]
  pitchFlag1/1 -> Multiport Switch2/1
  pitchFlag2/1 -> Multiport Switch2/2
  [AoA1] -> Multiport Switch2/3
  Multiport Switch2/1 -> AoA SP/1

== system FSCtrl_cl/FSCtrl/xcurrent-ellipse/pathFollowingControllerManta1/pathTrackingCtrl/Wrap Correction ==
  note: output = mod(input-pi,2*pi)-pi
      | wraps output to -pi to pi
      |
      | ex) 1.5*pi will become -.5pi
      | 	and -1.5pi will become .5pi
      |
      | to visualize, plot the fuction above
  u : Inport
  Add1 : Sum  Inputs=+-
  Add2 : Sum  Inputs=+-
  Constant1 : Constant  Value=pi
  Constant2 : Constant  Value=2*pi
  Constant3 : Constant  Value=pi
  Mod : Math  Operator=mod  SignedPower=on  SaturateOnIntegerOverflow=on
  y : Outport  VectorParamsAs1DForOutWhenUnconnected=off
  wires:
  u/1 -> Add1/1
  Constant1/1 -> Add1/2
  Add1/1 -> Mod/1
  Constant2/1 -> Mod/2
  Mod/1 -> Add2/1  "always_pos"
  Constant3/1 -> Add2/2
  Add2/1 -> y/1

== system FSCtrl_cl/FSCtrl/xcurrent-lemOfBooth/pathFollowingControllerManta/Lap Tracking/Subsystem ==
  note: this may have issues when it starts up after a hiatus for a multicycle spool in
      | Hopefully, it will work because the reasonable spooling ranges are already set
  S : Inport
  rst : Inport  Port=2
  AND : Logic  AllPortsSameDT=off  OutDataTypeStr=boolean
  Add : Sum
  Cast To Double : DataTypeConversion  OutDataTypeStr=double
  Compare To Constant : simulink/Logic and Bit Operations/Compare To Constant  relop=>=  const=.99  OutDataTypeStr=boolean
  Compare To Constant1 : simulink/Logic and Bit Operations/Compare To Constant  relop=<=  const=.01  OutDataTypeStr=boolean
  Divide : Product  Inputs=**
  Divide1 : Product  Inputs=**
  Gain : Gain  Gain=-1
  Max : MinMax  Function=max  Inputs=2
  Max1 : MinMax  Inputs=2
  One : Constant  OutDataTypeStr=Inherit: Inherit via back propagation
  Power : Math  Operator=pow  SaturateOnIntegerOverflow=on
  Power1 : Math  Operator=pow  SaturateOnIntegerOverflow=on
  memoryIC1 : Memory  InitialCondition=1
  memoryIC=0 : Memory
  memoryIC=1 : Memory  InitialCondition=1
  realLap : Outport
  wires:
  memoryIC1/1 -> Power/1
  memoryIC=1/1 -> Power1/1
  [zeroIfReset] -> Power1/2
  memoryIC=0/1 -> Divide1/1
  Divide1/1 -> Max/2
  [zeroIfReset] -> Divide1/2
  [zeroIfReset] -> Power/2
  [zeroIfReset] -> Divide/2
  AND/1 -> realLap/1
  Compare To Constant1/1 -> AND/2
  Compare To Constant/1 -> AND/1
  Cast To Double/1 -> Gain/1
  Power1/1 -> Max1/2
  Power/1 -> Max1/1
  Max/1 -> Compare To Constant/1, memoryIC=0/1
  Divide/1 -> Max/1
  One/1 -> Add/2
  Add/1 -> [zeroIfReset]
  Gain/1 -> Add/1
  S/1 -> memoryIC1/1, Divide/1
  rst/1 -> Cast To Double/1
  Max1/1 -> memoryIC=1/1, Compare To Constant1/1

== system FSCtrl_cl/FSCtrl/xcurrent-lemOfBooth/pathFollowingControllerManta/desiredMoment1/Subsystem ==
  Tthr : Inport
  vAppSqr : Inport  Port=2
  Add : Sum  Inputs=+-
  Constant : Constant  Value=pthCtrl1.Tmax.Value
  Divide : Product  Inputs=*/
  PID Controller : simulink/Continuous/PID Controller  Controller=PID  Form=Parallel  TimeDomain=Continuous-time  UseExternalTs=off  SampleTime=-1  IntegratorMethod=Forward Euler  FilterMethod=Forward Euler  ControllerParametersSource=internal  P=pthCtrl1.alphaCtrl.kp.Value  I=pthCtrl1.alphaCtrl.ki.Value  D=pthCtrl1.alphaCtrl.kd.Value  UseFilter=on  N=pthCtrl1.alphaCtrl.tau.Value  TunerSelectOption=Transfer Function Based (PID Tuner App)  InitialConditionSource=internal  InitialConditionForIntegrator=0  InitialConditionForFilter=0  DifferentiatorICPrevScaledInput=0  ExternalReset=none  TrackingMode=off  Kt=1  LimitOutput=on  UpperSaturationLimit=pthCtrl1.AoAConst.Value  LowerSaturationLimit=pthCtrl1.AoAmin.Value  LinearizeAsGain=on  AntiWindupMode=clamping  Kb=1  POutMin=[]  POutMax=[]  IOutMin=[]  IOutMax=[]  DOutMin=[]  DOutMax=[]  NOutMin=[]  NOutMax=[]  SumOutMin=[]  SumOutMax=[]  SaturationOutMin=[]  SaturationOutMax=[]  PParamMin=[]  PParamMax=[]  IParamMin=[]  IParamMax=[]  DParamMin=[]  DParamMax=[]  NParamMin=[]  NParamMax=[]  KbParamMin=[]  KbParamMax=[]  KtParamMin=[]  KtParamMax=[]  KbOutMin=[]  KbOutMax=[]  KtOutMin=[]  KtOutMax=[]  IntegratorOutMin=[]  IntegratorOutMax=[]  FilterOutMin=[]  FilterOutMax=[]  SumI1OutMin=[]  SumI1OutMax=[]  SumI2OutMin=[]  SumI2OutMax=[]  SumI3OutMin=[]  SumI3OutMax=[]  SumI4OutMin=[]  SumI4OutMax=[]  SumDOutMin=[]  SumDOutMax=[]  DifferentiatorOutMin=[]  DifferentiatorOutMax=[]  FilterDiffOutCoefMin=[]  FilterDiffOutCoefMax=[]  ReciprocalOutMin=[]  ReciprocalOutMax=[]  SumDenOutMin=[]  SumDenOutMax=[]  SumNumOutMin=[]  SumNumOutMax=[]  DivideOutMin=[]  DivideOutMax=[]  UdiffTsProdOutMin=[]  UdiffTsProdOutMax=[]  NTsProdOutMin=[]  NTsProdOutMax=[]  UintegralTsProdOutMin=[]  UintegralTsProdOutMax=[]  UngainTsProdOutMin=[]  UngainTsProdOutMax=[]  IntegratorContinuousStateAttributes=''  IntegratorStateMustResolveToSignalObject=off  IntegratorRTWStateStorageClass=Auto  FilterContinuousStateAttributes=''  FilterStateMustResolveToSignalObject=off  FilterRTWStateStorageClass=Auto  ParallelPVariant=InternalParameters  IdealPVariant=Disabled  IVariant=InternalParameters  DVariant=InternalParameters  IntegratorVariant=Continuous  SatVariant=Enabled  AWVariant=ContClampingParallel  PCopyVariant=Disabled  TRVariant=Disabled  FdbkBlocksVariant=Forward  IdealPFdbkVariant=Disabled  SatFdbkVariant=Disabled  DerivativeFilterVariant=ContFilter  NVariant=InternalParameters  NCopyVariant=Disabled  FilterICVariant=InternalICsFilter  IntegratorICVariant=InternalICs  ExternalResetVariant=Disabled  TRSumVariant=Passthrough  SumFdbkVariant=Disabled  SumVariant=Sum_PID  TsampFilterVariant=InternalTs  TsampNgainVariant=Passthrough  TsampIntegralVariant=Passthrough
  AoA SP : Outport
  wires:
  Divide/1 -> PID Controller/1  "TenErrNorm"
  Constant/1 -> Add/1  "maxTension"
  PID Controller/1 -> AoA SP/1
  Add/1 -> Divide/1  "TenErr"
  vAppSqr/1 -> Divide/2
  Tthr/1 -> Add/2  "thrTen"

== system FSCtrl_cl/FSCtrl/xcurrent-lemOfBooth/pathFollowingControllerManta/desiredMoment1/TangentRollCalculation ==
  note: Measuring tangent roll as the opposite
      | of the angle between the Body Y axis
      | and the tangent plane
  note: Angle between body Y and tangent Z
  note: Inverted because the right wing
      | being <90deg from Local down
      | is a negative roll about the +X axis
  note: Angle between body X and tangent Z
  tan2Gr : Inport
  bdy2Inert : Inport  Port=2
  Constant1 : Constant  Value=pi/2
  Constant2 : Constant  Value=pi/2
  Constant3 : Constant  Value=[0 1 0]'
  Constant4 : Constant  Value=[0 0 1]'
  Constant5 : Constant  Value=[1 0 0]'
  Constant6 : Constant  Value=[0 0 1]'
  Gain : Gain  Gain=-1
  Matrix Multiply{,1..3} (4 alike) : Product  Multiplication=Matrix(*)
  Subtract : Sum  Inputs=+-
  Subtract1 : Sum  Inputs=+-
  Terminator : Terminator
  angleBtw2DVecs : angleBtw2Vecs_ul/angleBtw2DVecs  SystemSampleTime=-1  Latency=0  AutoFrameSizeCalculation=off
  angleBtw2DVecs1 : Subsystem
  tanRoll : Outport  VectorParamsAs1DForOutWhenUnconnected=off
  wires:
  Subtract/1 -> Gain/1
  Constant3/1 -> Matrix Multiply/2
  angleBtw2DVecs/1 -> Subtract/2
  Constant2/1 -> Subtract/1
  Matrix Multiply1/1 -> angleBtw2DVecs/1
  Constant4/1 -> Matrix Multiply1/2
  Matrix Multiply/1 -> angleBtw2DVecs/2
  Gain/1 -> tanRoll/1  "tanRoll"
  bdy2Inert/1 -> Matrix Multiply2/1, Matrix Multiply/1
  Subtract1/1 -> Terminator/1  "tanPitch"
  tan2Gr/1 -> Matrix Multiply3/1, Matrix Multiply1/1
  Matrix Multiply2/1 -> angleBtw2DVecs1/2(vec2)
  Constant6/1 -> Matrix Multiply3/2
  Matrix Multiply3/1 -> angleBtw2DVecs1/1(vec1)
  Constant1/1 -> Subtract1/1
  angleBtw2DVecs1/1(angle) -> Subtract1/2
  Constant5/1 -> Matrix Multiply2/2

== system FSCtrl_cl/FSCtrl/xcurrent-lemOfBooth/pathFollowingControllerManta/desiredMoment1/Wrap Correction ==
  note: output = mod(input-pi,2*pi)-pi
      | wraps output to -pi to pi
      |
      | ex) 1.5*pi will become -.5pi
      | 	and -1.5pi will become .5pi
      |
      | to visualize, plot the fuction above
  u : Inport
  Add1 : Sum  Inputs=+-
  Add2 : Sum  Inputs=+-
  Constant1 : Constant  Value=pi
  Constant2 : Constant  Value=2*pi
  Constant3 : Constant  Value=pi
  Mod : Math  Operator=mod  SignedPower=on  SaturateOnIntegerOverflow=on
  y : Outport  VectorParamsAs1DForOutWhenUnconnected=off
  wires:
  u/1 -> Add1/1
  Constant1/1 -> Add1/2
  Add1/1 -> Mod/1
  Constant2/1 -> Mod/2
  Mod/1 -> Add2/1  "always_pos"
  Constant3/1 -> Add2/2
  Add2/1 -> y/1

== system FSCtrl_cl/FSCtrl/xcurrent-lemOfBooth/pathFollowingControllerManta/desiredMoment1/filteredPIDController4 ==
  u : Inport  PortDimensions=1
  Add : Sum  Inputs=+-
  Add1 : Sum  Inputs=+++
  Divide : Product  Inputs=*/
  Integrator : Integrator
  Integrator1 : Integrator
  Integrator2 : Integrator
  Max : MinMax  Function=max  Inputs=2
  Weighted Sample Time : SampleTimeMath  TsampMathOp=Ts Only
  const : Constant
  kd : Gain  Gain=kd
  ki : Gain  Gain=ki
  kp : Gain  Gain=kp
  tau : Constant  Value=Value
  y : Outport  PortDimensions=1  VectorParamsAs1DForOutWhenUnconnected=off
  wires:
  u/1 -> [u]
  kp/1 -> Add/1
  [y] -> Add/2
  Add/1 -> Integrator/1
  [u] -> kp/1
  Max/1 -> Divide/2
  tau/1 -> Max/2
  Integrator1/1 -> Integrator2/1
  ki/1 -> Integrator1/1
  [u] -> ki/1
  [u] -> kd/1
  Integrator2/1 -> Add1/2
  Integrator/1 -> Add1/1
  kd/1 -> Add1/3
  Add1/1 -> Divide/1
  Divide/1 -> [y], y/1
  Weighted Sample Time/1 -> Max/1
  const/1 -> Weighted Sample Time/1

== system FSCtrl_cl/FSCtrl/non-xcurrent/LaRController/desiredMoment/TangentRollCalculation/angleBtw2DVecs1 ==
  vec1 : Inport
  vec2 : Inport  Port=2
  Abs : Abs
  Atan2 : Trigonometry  Operator=atan2
  Cross Product : vrlib/Utilities/Cross Product
      settings: SourceProductBaseCode=VR
  Dot Product : DotProduct  InputSameDT=on  OutDataTypeStr=Inherit: Inherit via internal rule
  Dot Product1 : DotProduct  InputSameDT=on  OutDataTypeStr=Inherit: Inherit via internal rule
  Sqrt : Sqrt  SaturateOnIntegerOverflow=on
  angle : Outport  VectorParamsAs1DForOutWhenUnconnected=off
  wires:
  Sqrt/1 -> Atan2/1
  Dot Product1/1 -> Sqrt/1
  Abs/1 -> angle/1
  Dot Product/1 -> Atan2/2
  Cross Product/1 -> Dot Product1/2, Dot Product1/1
  vec2/1 -> Dot Product/2, Cross Product/1
  vec1/1 -> Cross Product/2, Dot Product/1
  Atan2/1 -> Abs/1

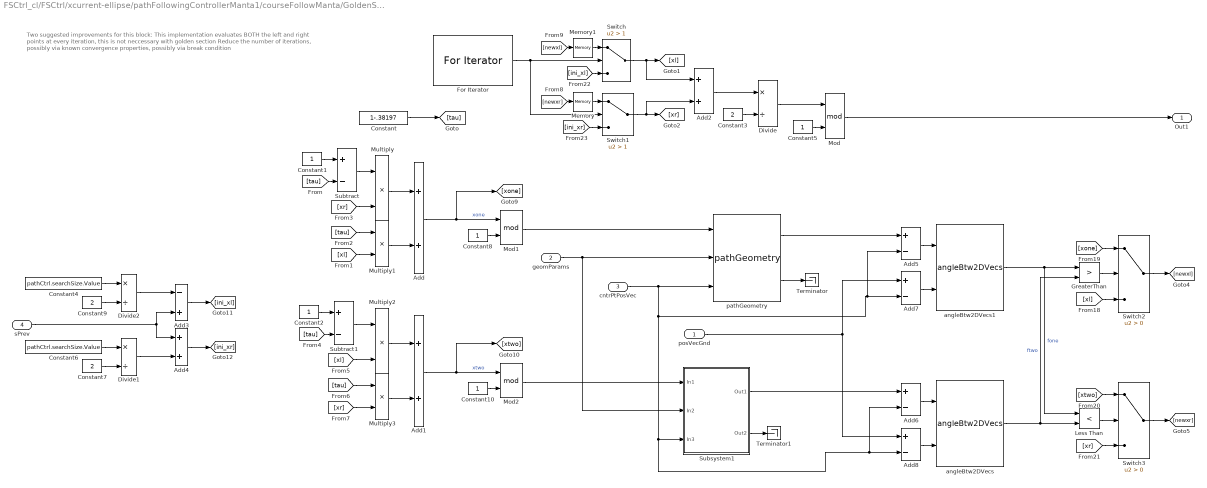
== system FSCtrl_cl/FSCtrl/xcurrent-ellipse/pathFollowingControllerManta1/courseFollowManta/GoldenSectionPathSearch/GoldenSectionSimulink ==
  note: Two suggested improvements for this block:
      | This implementation evaluates BOTH the left and right points at every iteration, this is not neccessary with golden section
      | Reduce the number of iterations, possibly via known convergence properties, possibly via break condition
  posVecGnd : Inport
  geomParams : Inport  Port=2
  cntrPtPosVec : Inport  Port=3
  sPrev : Inport  Port=4
  Add{,1..2,4} (4 alike) : Sum
  Add3 : Sum  Inputs=-+
  Add{5..8} (4 alike) : Sum  Inputs=+-
  Constant : Constant  Value=1-.38197
  Constant{1..2,5,8,10} (5 alike) : Constant
  Constant3 : Constant  Value=2
  Constant4 : Constant  Value=pathCtrl.searchSize.Value
  Constant6 : Constant  Value=pathCtrl.searchSize.Value
  Constant7 : Constant  Value=2
  Constant9 : Constant  Value=2
  Divide : Product  Inputs=*/
  Divide1 : Product  Inputs=*/
  Divide2 : Product  Inputs=*/
  For Iterator : ForIterator  IterationLimit=25
  GreaterThan : RelationalOperator  Operator=>  OutDataTypeStr=boolean  RndMeth=Simplest
  Less Than : RelationalOperator  Operator=<  OutDataTypeStr=boolean  RndMeth=Simplest
  Memory : Memory  InheritSampleTime=on
  Memory1 : Memory  InheritSampleTime=on
  Mod : Math  Operator=mod  SignedPower=on  SaturateOnIntegerOverflow=on
  Mod1 : Math  Operator=mod  SignedPower=on  SaturateOnIntegerOverflow=on
  Mod2 : Math  Operator=mod  SignedPower=on  SaturateOnIntegerOverflow=on
  Multiply{,1..3} (4 alike) : Product
  Subsystem1 : Subsystem
  Subtract : Sum  Inputs=+-
  Subtract1 : Sum  Inputs=+-
  Switch : Switch  Criteria=u2 > Threshold  Threshold=1
  Switch1 : Switch  Criteria=u2 > Threshold  Threshold=1
  Switch2 : Switch  Criteria=u2 > Threshold
  Switch3 : Switch  Criteria=u2 > Threshold
  Terminator : Terminator
  Terminator1 : Terminator
  angleBtw2DVecs : angleBtw2Vecs_ul/angleBtw2DVecs  SystemSampleTime=-1  Latency=0  AutoFrameSizeCalculation=off
  angleBtw2DVecs1 : angleBtw2Vecs_ul/angleBtw2DVecs  SystemSampleTime=-1  Latency=0  AutoFrameSizeCalculation=off
  pathGeometry : pathGeometry_ul/pathGeometry  SystemSampleTime=-1  Latency=0  AutoFrameSizeCalculation=off
  Out1 : Outport
  wires:
  Add8/1 -> angleBtw2DVecs/2
  Multiply1/1 -> Add/2
  Switch3/1 -> [newxr]
  [ini_xl] -> Switch/3
  Mod/1 -> Out1/1
  Divide2/1 -> Add3/1
  Switch2/1 -> [newxl]
  pathGeometry/2 -> Terminator/1
  [newxl] -> Memory1/1
  Constant6/1 -> Divide1/1
  Add6/1 -> angleBtw2DVecs/1
  Constant10/1 -> Mod2/2
  Add2/1 -> Divide/1
  [xl] -> Switch2/3
  [xr] -> Switch3/3
  Divide/1 -> Mod/1
  [xl] -> Multiply2/2
  Multiply3/1 -> Add1/2
  Add5/1 -> angleBtw2DVecs1/1
  sPrev/1 -> Add3/2, Add4/1
  Less Than/1 -> Switch3/2
  Constant3/1 -> Divide/2
  Add4/1 -> [ini_xr]
  Constant9/1 -> Divide2/2
  [xr] -> Multiply/2
  Add3/1 -> [ini_xl]
  Divide1/1 -> Add4/2
  Mod1/1 -> pathGeometry/1
  Memory/1 -> Switch1/1
  [newxr] -> Memory/1
  Add7/1 -> angleBtw2DVecs1/2
  [tau] -> Multiply1/1
  [xone] -> Switch2/1
  [ini_xr] -> Switch1/3
  angleBtw2DVecs1/1 -> GreaterThan/1, Less Than/1  "fone"
  Constant4/1 -> Divide2/1
  Mod2/1 -> Subsystem1/1(In1)
  Multiply2/1 -> Add1/1
  Switch1/1 -> [xr], Add2/2
  Constant/1 -> [tau]
  Add/1 -> Mod1/1, [xone]  "xone"
  For Iterator/1 -> Switch/2, Switch1/2
  Memory1/1 -> Switch/1
  [tau] -> Multiply3/1
  [tau] -> Subtract/2
  [xtwo] -> Switch3/1
  Multiply/1 -> Add/1
  [xl] -> Multiply1/2
  Subsystem1/2(Out2) -> Terminator1/1
  Subtract/1 -> Multiply/1
  Constant7/1 -> Divide1/2
  Add1/1 -> Mod2/1, [xtwo]  "xtwo"
  [tau] -> Subtract1/2
  angleBtw2DVecs/1 -> Less Than/2, GreaterThan/2  "ftwo"
  Constant5/1 -> Mod/2
  Constant1/1 -> Subtract/1
  posVecGnd/1 -> Add7/1, Add8/1
  GreaterThan/1 -> Switch2/2
  pathGeometry/1 -> Add5/1
  Constant8/1 -> Mod1/2
  [xr] -> Multiply3/2
  Subsystem1/1(Out1) -> Add6/1
  Constant2/1 -> Subtract1/1
  geomParams/1 -> Subsystem1/2(In2), pathGeometry/2
  Switch/1 -> [xl], Add2/1
  cntrPtPosVec/1 -> pathGeometry/3, Add7/2, Add5/2, Subsystem1/3(In3), Add8/2, Add6/2
  Subtract1/1 -> Multiply2/1

== system FSCtrl_cl/FSCtrl/xcurrent-ellipse/pathFollowingControllerManta1/pathTrackingCtrl/TangentRollCalculation/angleBtw2DVecs1 ==
  vec1 : Inport
  vec2 : Inport  Port=2
  Abs : Abs
  Atan2 : Trigonometry  Operator=atan2
  Cross Product : vrlib/Utilities/Cross Product
      settings: SourceProductBaseCode=VR
  Dot Product : DotProduct  InputSameDT=on  OutDataTypeStr=Inherit: Inherit via internal rule
  Dot Product1 : DotProduct  InputSameDT=on  OutDataTypeStr=Inherit: Inherit via internal rule
  Sqrt : Sqrt  SaturateOnIntegerOverflow=on
  angle : Outport  VectorParamsAs1DForOutWhenUnconnected=off
  wires:
  Atan2/1 -> Abs/1
  vec1/1 -> Dot Product/1, Cross Product/2
  vec2/1 -> Cross Product/1, Dot Product/2
  Cross Product/1 -> Dot Product1/1, Dot Product1/2
  Dot Product/1 -> Atan2/2
  Abs/1 -> angle/1
  Dot Product1/1 -> Sqrt/1
  Sqrt/1 -> Atan2/1

== system FSCtrl_cl/FSCtrl/xcurrent-lemOfBooth/pathFollowingControllerManta/desiredMoment1/TangentRollCalculation/angleBtw2DVecs1 ==
  vec1 : Inport
  vec2 : Inport  Port=2
  Abs : Abs
  Atan2 : Trigonometry  Operator=atan2
  Cross Product : vrlib/Utilities/Cross Product
      settings: SourceProductBaseCode=VR
  Dot Product : DotProduct  InputSameDT=on  OutDataTypeStr=Inherit: Inherit via internal rule
  Dot Product1 : DotProduct  InputSameDT=on  OutDataTypeStr=Inherit: Inherit via internal rule
  Sqrt : Sqrt  SaturateOnIntegerOverflow=on
  angle : Outport  VectorParamsAs1DForOutWhenUnconnected=off
  wires:
  Atan2/1 -> Abs/1
  vec1/1 -> Dot Product/1, Cross Product/2
  vec2/1 -> Cross Product/1, Dot Product/2
  Cross Product/1 -> Dot Product1/1, Dot Product1/2
  Dot Product/1 -> Atan2/2
  Abs/1 -> angle/1
  Dot Product1/1 -> Sqrt/1
  Sqrt/1 -> Atan2/1

== system FSCtrl_cl/FSCtrl/xcurrent-ellipse/pathFollowingControllerManta1/courseFollowManta/GoldenSectionPathSearch/GoldenSectionSimulink/Subsystem1 ==
  In1 : Inport
  In2 : Inport  Port=2
  In3 : Inport  Port=3
  pathGeometry : pathGeometry_ul/pathGeometry  SystemSampleTime=-1  Latency=0  AutoFrameSizeCalculation=off
  Out1 : Outport  VectorParamsAs1DForOutWhenUnconnected=off
  Out2 : Outport  Port=2  VectorParamsAs1DForOutWhenUnconnected=off
  wires:
  pathGeometry/2 -> Out2/1
  In1/1 -> pathGeometry/1
  In3/1 -> pathGeometry/3
  pathGeometry/1 -> Out1/1
  In2/1 -> pathGeometry/2

== matlab function FSCtrl_cl/FSCtrl/non-xcurrent/LaRController/winchController/MATLAB Function ==
  data: thrLength input; thrTension input; posAng input; Ctrl output; eulAng input; coneWidth parameter; spd parameter; elevSP input; thrSP input; minTen parameter; time input
function Ctrl  = fcn(thrLength, thrTension, posAng, eulAng, coneWidth,  spd, elevSP, thrSP, minTen, time)

Ctrl  = winchCtrl(thrLength, thrTension, posAng, eulAng, coneWidth,  spd, elevSP, thrSP, minTen, time);
